simulink model "LugreFrictionTester"  (R2023b)
settings: Solver=ode4  StartTime=0.0  StopTime=t_final(end)  FixedStep=1e-3  RelTol=1e-3
undefined symbols (not defined in the file or in its folder): Aeff, m, xc, xc_dot
settings Model: Creator=snr  LastModifiedBy=snr

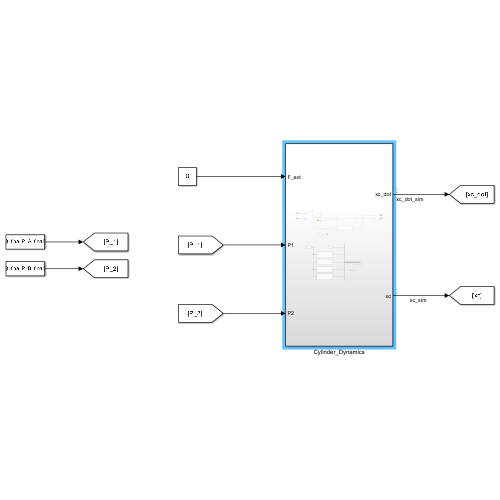
[thumbnail: Simulink's stored preview of the top-level diagram]
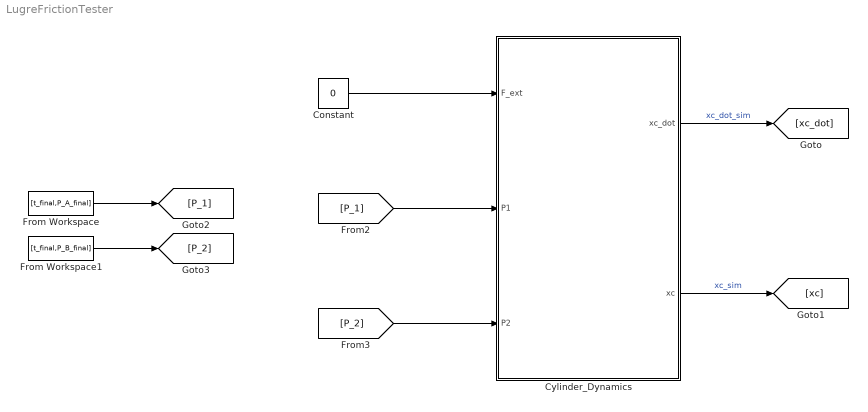
== system LugreFrictionTester ==
  Constant : Constant  Value=0  OutDataTypeStr=double
  Cylinder_Dynamics : Subsystem
  From Workspace : FromWorkspace  VariableName=[t_final,P_A_final]
  From Workspace1 : FromWorkspace  VariableName=[t_final,P_B_final]
  wires:
  Constant/1 -> Cylinder_Dynamics/1(F_ext)
  Cylinder_Dynamics/2(xc) -> [xc]  "xc_sim"
  [P_2] -> Cylinder_Dynamics/3(P2)
  [P_1] -> Cylinder_Dynamics/2(P1)
  Cylinder_Dynamics/1(xc_dot) -> [xc_dot]  "xc_dot_sim"
  From Workspace/1 -> [P_1]
  From Workspace1/1 -> [P_2]

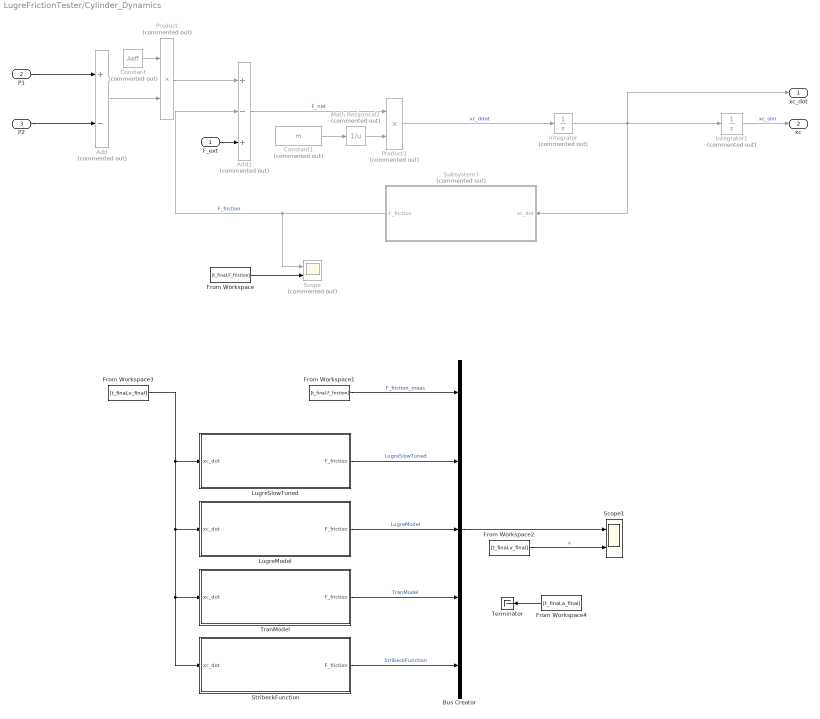
== system LugreFrictionTester/Cylinder_Dynamics ==
  F_ext : Inport  OutDataTypeStr=double
  P1 : Inport  Port=2  OutDataTypeStr=double
  P2 : Inport  Port=3  OutDataTypeStr=double
  Add : Sum  Commented=on  Inputs=+-
  Add1 : Sum  Commented=on  Inputs=+-+
  Bus Creator : BusCreator  Inputs=5
  Constant : Constant  Commented=on  Value=Aeff  OutDataTypeStr=double
  Constant1 : Constant  Commented=on  Value=m  OutDataTypeStr=double
  From Workspace : FromWorkspace  VariableName=[t_final,F_friction]
  From Workspace1 : FromWorkspace  VariableName=[t_final,F_friction]
  From Workspace2 : FromWorkspace  VariableName=[t_final,v_final]
  From Workspace3 : FromWorkspace  VariableName=[t_final,v_final]
  From Workspace4 : FromWorkspace  VariableName=[t_final,a_final]
  Integrator : Integrator  Commented=on  InitialCondition=xc_dot(1)
  Integrator1 : Integrator  Commented=on  InitialCondition=xc(1)
  LugreModel : Subsystem
  LugreSlowTuned : Subsystem
  Math Reciprocal2 : Math  Commented=on  Operator=reciprocal  SignedPower=on
  Product : Product  Commented=on
  Product1 : Product  Commented=on
  Scope : Scope  Commented=on  NumInputPorts=2
  Scope1 : Scope  NumInputPorts=2
  StribeckFunction : Subsystem
  Subsystem3 : Subsystem  Commented=on
  Terminator : Terminator
  TranModel : Subsystem
  xc_dot : Outport  OutDataTypeStr=double
  xc : Outport  Port=2  OutDataTypeStr=double
  wires:
  P2/1 -> Add/2
  P1/1 -> Add/1
  F_ext/1 -> Add1/3
  Integrator1/1 -> xc/1  "xc_sim"
  Add/1 -> Product/2
  Constant/1 -> Product/1
  Add1/1 -> Product1/1  "F_net"
  Constant1/1 -> Math Reciprocal2/1
  Math Reciprocal2/1 -> Product1/2
  Product1/1 -> Integrator/1  "xc_ddot"
  Integrator/1 -> Subsystem3/1(xc_dot), xc_dot/1, Integrator1/1
  Subsystem3/1(F_friction) -> Scope/1, Add1/2  "F_friction"
  Product/1 -> Add1/1
  From Workspace/1 -> Scope/2
  From Workspace3/1 -> StribeckFunction/1(xc_dot), TranModel/1(xc_dot), LugreModel/1(xc_dot), LugreSlowTuned/1(xc_dot)
  LugreModel/1(F_friction) -> Bus Creator/3  "LugreModel"
  TranModel/1(F_friction) -> Bus Creator/4  "TranModel"
  StribeckFunction/1(F_friction) -> Bus Creator/5  "StribeckFunction"
  From Workspace1/1 -> Bus Creator/1  "F_friction_meas"
  Bus Creator/1 -> Scope1/1
  From Workspace2/1 -> Scope1/2  "v"
  LugreSlowTuned/1(F_friction) -> Bus Creator/2  "LugreSlowTuned"
  From Workspace4/1 -> Terminator/1

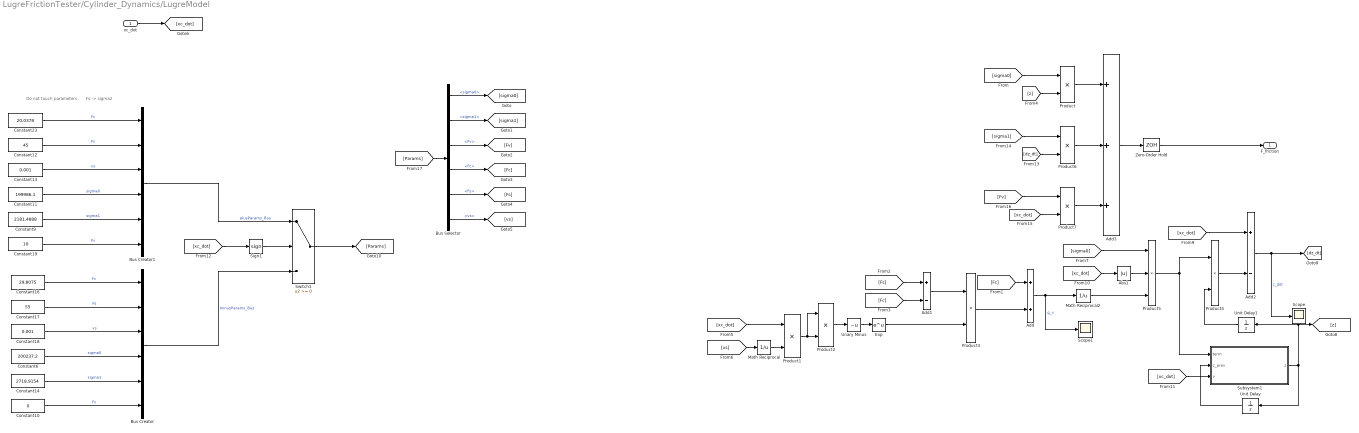
== system LugreFrictionTester/Cylinder_Dynamics/LugreModel ==
  note: Do not touch parameters
  note: Fv -> sigma2
  xc_dot : Inport
  Abs1 : Abs  SaturateOnIntegerOverflow=off
  Add : Sum
  Add1 : Sum  Inputs=+-
  Add2 : Sum  Inputs=+-
  Add3 : Sum  Inputs=+++
  Bus Selector : BusSelector  OutputSignals=sigma0,sigma1,Fv,Fc,Fs,vs
  Bus Creator : BusCreator  Inputs=6
  Bus Creator1 : BusCreator  Inputs=6
  Constant10 : Constant  Value=0  OutDataTypeStr=double
  Constant11 : Constant  Value=199986.1  OutDataTypeStr=double
  Constant12 : Constant  Value=45  OutDataTypeStr=double
  Constant13 : Constant  Value=0.001  OutDataTypeStr=double
  Constant14 : Constant  Value=2718.9154  OutDataTypeStr=double
  Constant16 : Constant  Value=29.8075  OutDataTypeStr=double
  Constant17 : Constant  Value=55  OutDataTypeStr=double
  Constant18 : Constant  Value=0.001  OutDataTypeStr=double
  Constant19 : Constant  Value=10  OutDataTypeStr=double
  Constant23 : Constant  Value=20.0378  OutDataTypeStr=double
  Constant6 : Constant  Value=200237.2  OutDataTypeStr=double
  Constant9 : Constant  Value=2181.4888  OutDataTypeStr=double
  Exp : Math  SignedPower=on
  Math Reciprocal : Math  Operator=reciprocal  SignedPower=on
  Math Reciprocal2 : Math  Operator=reciprocal  SignedPower=on
  Product{,1..4,6..7} (7 alike) : Product
  Product5 : Product  Inputs=3
  Scope : Scope
  Scope1 : Scope
  Sign1 : Signum
  Subsystem1 : Subsystem
  Switch1 : Switch  SaturateOnIntegerOverflow=off  InputSameDT=off
  Unary Minus : UnaryMinus
  Unit Delay : UnitDelay  SampleTime=-1  HasFrameUpgradeWarning=on
  Unit Delay1 : UnitDelay  SampleTime=-1  HasFrameUpgradeWarning=on
  Zero-Order Hold : ZeroOrderHold  SampleTime=1e-3
  F_friction : Outport
  wires:
  Zero-Order Hold/1 -> F_friction/1
  Product4/1 -> Add2/2
  Product5/1 -> Product4/1, Subsystem1/1(term)
  Unit Delay/1 -> Subsystem1/2(z_prev)
  Subsystem1/1(z) -> Unit Delay/1, Unit Delay1/1, [z]
  [xc_dot] -> Subsystem1/3(v)
  Unit Delay1/1 -> Product4/2
  [xc_dot] -> Add2/1
  Sign1/1 -> Switch1/2
  Add2/1 -> [dz_dt], Scope/1  "z_dot"
  Exp/1 -> Product3/2
  xc_dot/1 -> [xc_dot]
  Math Reciprocal2/1 -> Product5/3
  Bus Selector/6 -> [vs]  "<vs>"
  Bus Selector/5 -> [Fs]  "<Fs>"
  Bus Selector/4 -> [Fc]  "<Fc>"
  Bus Selector/3 -> [Fv]  "<Fv>"
  Bus Selector/2 -> [sigma1]  "<sigma1>"
  Bus Selector/1 -> [sigma0]  "<sigma0>"
  [Params] -> Bus Selector/1
  Switch1/1 -> [Params]
  Bus Creator/1 -> Switch1/3  "minusParams_Bus"
  Bus Creator1/1 -> Switch1/1  "plusParams_Bus"
  [xc_dot] -> Sign1/1
  Product3/1 -> Add/2
  [sigma0] -> Product/1
  [Fc] -> Add/1
  [Fs] -> Add1/1
  [Fc] -> Add1/2
  [vs] -> Math Reciprocal/1
  Math Reciprocal/1 -> Product1/2
  [xc_dot] -> Product1/1
  Product1/1 -> Product2/1, Product2/2
  Product2/1 -> Unary Minus/1
  Unary Minus/1 -> Exp/1
  Add1/1 -> Product3/1
  [xc_dot] -> Abs1/1
  Add/1 -> Scope1/1, Math Reciprocal2/1  "g_v"
  Abs1/1 -> Product5/2
  [sigma0] -> Product5/1
  [z] -> Product/2
  Product/1 -> Add3/1
  [sigma1] -> Product6/1
  [dz_dt] -> Product6/2
  [xc_dot] -> Product7/2
  [Fv] -> Product7/1
  Product6/1 -> Add3/2
  Product7/1 -> Add3/3
  Add3/1 -> Zero-Order Hold/1
  Constant23/1 -> Bus Creator1/1  "Fc"
  Constant19/1 -> Bus Creator1/6  "Fv"
  Constant11/1 -> Bus Creator1/4  "sigma0"
  Constant9/1 -> Bus Creator1/5  "sigma1"
  Constant16/1 -> Bus Creator/1  "Fc"
  Constant10/1 -> Bus Creator/6  "Fv"
  Constant6/1 -> Bus Creator/4  "sigma0"
  Constant14/1 -> Bus Creator/5  "sigma1"
  Constant17/1 -> Bus Creator/2  "Fs"
  Constant12/1 -> Bus Creator1/2  "Fs"
  Constant13/1 -> Bus Creator1/3  "vs"
  Constant18/1 -> Bus Creator/3  "vs"

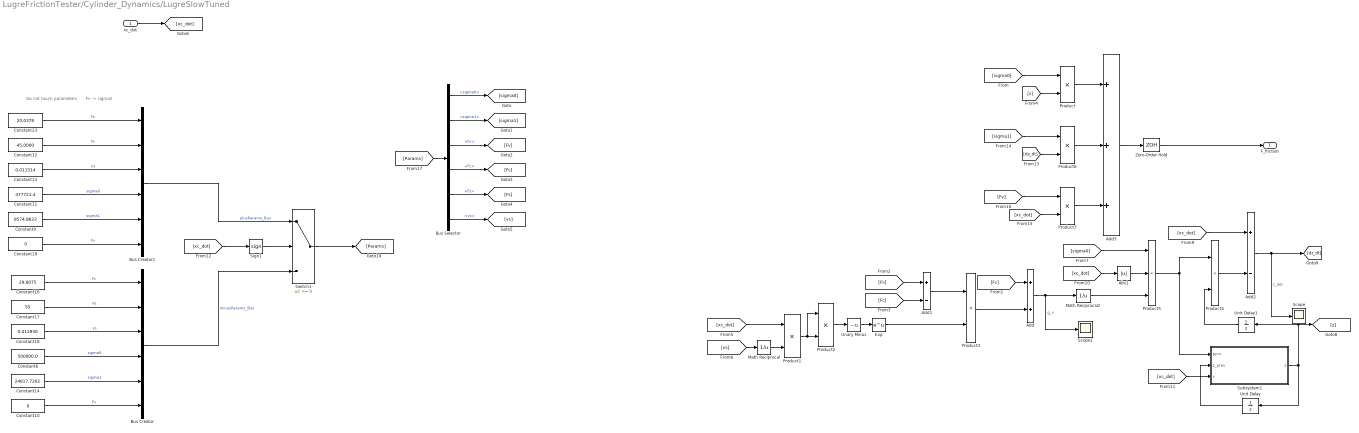
== system LugreFrictionTester/Cylinder_Dynamics/LugreSlowTuned ==
  note: Fv -> sigma2
  note: Do not touch parameters
  xc_dot : Inport
  Abs1 : Abs  SaturateOnIntegerOverflow=off
  Add : Sum
  Add1 : Sum  Inputs=+-
  Add2 : Sum  Inputs=+-
  Add3 : Sum  Inputs=+++
  Bus Selector : BusSelector  OutputSignals=sigma0,sigma1,Fv,Fc,Fs,vs
  Bus Creator : BusCreator  Inputs=6
  Bus Creator1 : BusCreator  Inputs=6
  Constant10 : Constant  Value=0  OutDataTypeStr=double
  Constant11 : Constant  Value=477721.4  OutDataTypeStr=double
  Constant12 : Constant  Value=45.0000  OutDataTypeStr=double
  Constant13 : Constant  Value=0.011514  OutDataTypeStr=double
  Constant14 : Constant  Value=24817.7202  OutDataTypeStr=double
  Constant16 : Constant  Value=29.8075  OutDataTypeStr=double
  Constant17 : Constant  Value=55  OutDataTypeStr=double
  Constant18 : Constant  Value=0.012930  OutDataTypeStr=double
  Constant19 : Constant  Value=0  OutDataTypeStr=double
  Constant23 : Constant  Value=20.0378  OutDataTypeStr=double
  Constant6 : Constant  Value=500000.0  OutDataTypeStr=double
  Constant9 : Constant  Value=8574.8623  OutDataTypeStr=double
  Exp : Math  SignedPower=on
  Math Reciprocal : Math  Operator=reciprocal  SignedPower=on
  Math Reciprocal2 : Math  Operator=reciprocal  SignedPower=on
  Product{,1..4,6..7} (7 alike) : Product
  Product5 : Product  Inputs=3
  Scope : Scope
  Scope1 : Scope
  Sign1 : Signum
  Subsystem1 : Subsystem
  Switch1 : Switch  SaturateOnIntegerOverflow=off  InputSameDT=off
  Unary Minus : UnaryMinus
  Unit Delay : UnitDelay  SampleTime=-1  HasFrameUpgradeWarning=on
  Unit Delay1 : UnitDelay  SampleTime=-1  HasFrameUpgradeWarning=on
  Zero-Order Hold : ZeroOrderHold  SampleTime=1e-3
  F_friction : Outport
  wires:
  Constant18/1 -> Bus Creator/3  "vs"
  Constant13/1 -> Bus Creator1/3  "vs"
  Constant12/1 -> Bus Creator1/2  "Fs"
  Constant17/1 -> Bus Creator/2  "Fs"
  Constant14/1 -> Bus Creator/5  "sigma1"
  Constant6/1 -> Bus Creator/4  "sigma0"
  Constant10/1 -> Bus Creator/6  "Fv"
  Constant16/1 -> Bus Creator/1  "Fc"
  Constant9/1 -> Bus Creator1/5  "sigma1"
  Constant11/1 -> Bus Creator1/4  "sigma0"
  Constant19/1 -> Bus Creator1/6  "Fv"
  Constant23/1 -> Bus Creator1/1  "Fc"
  Add3/1 -> Zero-Order Hold/1
  Product7/1 -> Add3/3
  Product6/1 -> Add3/2
  [Fv] -> Product7/1
  [xc_dot] -> Product7/2
  [dz_dt] -> Product6/2
  [sigma1] -> Product6/1
  Product/1 -> Add3/1
  [z] -> Product/2
  [sigma0] -> Product5/1
  Abs1/1 -> Product5/2
  Add/1 -> Math Reciprocal2/1, Scope1/1  "g_v"
  [xc_dot] -> Abs1/1
  Add1/1 -> Product3/1
  Unary Minus/1 -> Exp/1
  Product2/1 -> Unary Minus/1
  Product1/1 -> Product2/2, Product2/1
  [xc_dot] -> Product1/1
  Math Reciprocal/1 -> Product1/2
  [vs] -> Math Reciprocal/1
  [Fc] -> Add1/2
  [Fs] -> Add1/1
  [Fc] -> Add/1
  [sigma0] -> Product/1
  Product3/1 -> Add/2
  [xc_dot] -> Sign1/1
  Bus Creator1/1 -> Switch1/1  "plusParams_Bus"
  Bus Creator/1 -> Switch1/3  "minusParams_Bus"
  Switch1/1 -> [Params]
  [Params] -> Bus Selector/1
  Bus Selector/1 -> [sigma0]  "<sigma0>"
  Bus Selector/2 -> [sigma1]  "<sigma1>"
  Bus Selector/3 -> [Fv]  "<Fv>"
  Bus Selector/4 -> [Fc]  "<Fc>"
  Bus Selector/5 -> [Fs]  "<Fs>"
  Bus Selector/6 -> [vs]  "<vs>"
  Math Reciprocal2/1 -> Product5/3
  xc_dot/1 -> [xc_dot]
  Exp/1 -> Product3/2
  Add2/1 -> Scope/1, [dz_dt]  "z_dot"
  Sign1/1 -> Switch1/2
  [xc_dot] -> Add2/1
  Unit Delay1/1 -> Product4/2
  [xc_dot] -> Subsystem1/3(v)
  Subsystem1/1(z) -> [z], Unit Delay1/1, Unit Delay/1
  Unit Delay/1 -> Subsystem1/2(z_prev)
  Product5/1 -> Subsystem1/1(term), Product4/1
  Product4/1 -> Add2/2
  Zero-Order Hold/1 -> F_friction/1

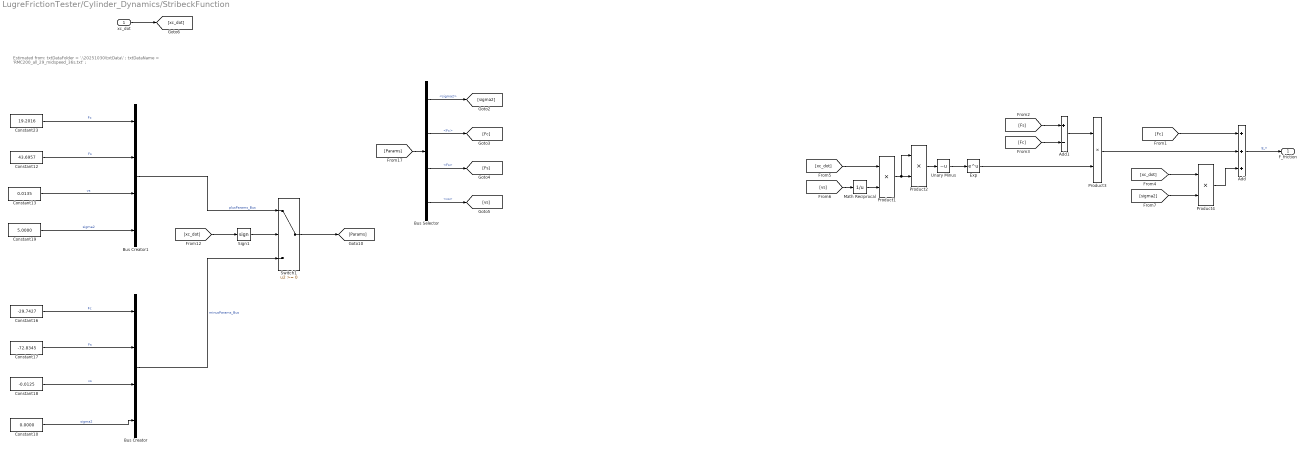
== system LugreFrictionTester/Cylinder_Dynamics/StribeckFunction ==
  note: Estimated from:
      |
      | txtDataFolder = '.\20251030\txtData\' ;
      | txtDataName = 'RMC200_all_29_midspeed_36s.txt' ;
  xc_dot : Inport
  Add : Sum  Inputs=+++
  Add1 : Sum  Inputs=+-
  Bus Selector : BusSelector  OutputSignals=sigma2,Fc,Fs,vs
  Bus Creator : BusCreator  Inputs=4
  Bus Creator1 : BusCreator  Inputs=4
  Constant10 : Constant  Value=0.0000  OutDataTypeStr=double
  Constant12 : Constant  Value=43.6957  OutDataTypeStr=double
  Constant13 : Constant  Value=0.0135  OutDataTypeStr=double
  Constant16 : Constant  Value=-29.7427  OutDataTypeStr=double
  Constant17 : Constant  Value=-72.8345  OutDataTypeStr=double
  Constant18 : Constant  Value=-0.0125  OutDataTypeStr=double
  Constant19 : Constant  Value=5.0000  OutDataTypeStr=double
  Constant23 : Constant  Value=19.2016  OutDataTypeStr=double
  Exp : Math  SignedPower=on
  Math Reciprocal : Math  Operator=reciprocal  SignedPower=on
  Product{1..4} (4 alike) : Product
  Sign1 : Signum
  Switch1 : Switch  SaturateOnIntegerOverflow=off  InputSameDT=off
  Unary Minus : UnaryMinus
  F_friction : Outport
  wires:
  Sign1/1 -> Switch1/2
  Exp/1 -> Product3/2
  xc_dot/1 -> [xc_dot]
  Bus Selector/4 -> [vs]  "<vs>"
  Bus Selector/3 -> [Fs]  "<Fs>"
  Bus Selector/2 -> [Fc]  "<Fc>"
  Bus Selector/1 -> [sigma2]  "<sigma2>"
  [Params] -> Bus Selector/1
  Switch1/1 -> [Params]
  Bus Creator/1 -> Switch1/3  "minusParams_Bus"
  Bus Creator1/1 -> Switch1/1  "plusParams_Bus"
  [xc_dot] -> Sign1/1
  Product3/1 -> Add/2
  [Fc] -> Add/1
  [Fs] -> Add1/1
  [Fc] -> Add1/2
  [vs] -> Math Reciprocal/1
  Math Reciprocal/1 -> Product1/2
  [xc_dot] -> Product1/1
  Product1/1 -> Product2/1, Product2/2
  Product2/1 -> Unary Minus/1
  Unary Minus/1 -> Exp/1
  Add1/1 -> Product3/1
  Add/1 -> F_friction/1  "g_v"
  Constant23/1 -> Bus Creator1/1  "Fc"
  Constant19/1 -> Bus Creator1/4  "sigma2"
  Constant16/1 -> Bus Creator/1  "Fc"
  Constant10/1 -> Bus Creator/4  "sigma2"
  Constant17/1 -> Bus Creator/2  "Fs"
  Constant12/1 -> Bus Creator1/2  "Fs"
  Constant13/1 -> Bus Creator1/3  "vs"
  Constant18/1 -> Bus Creator/3  "vs"
  [xc_dot] -> Product4/1
  [sigma2] -> Product4/2
  Product4/1 -> Add/3

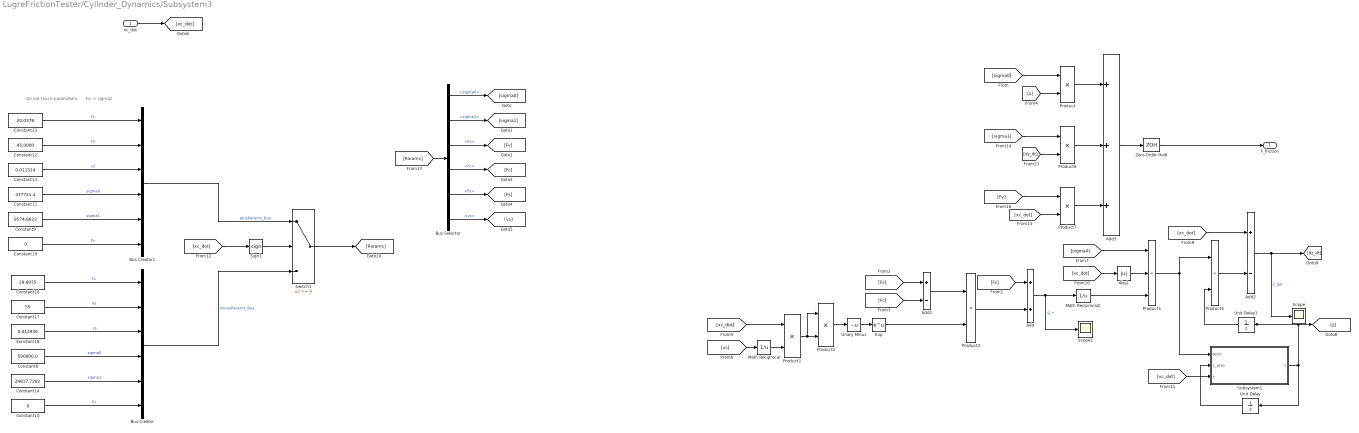
== system LugreFrictionTester/Cylinder_Dynamics/Subsystem3 ==
  note: Do not touch parameters
  note: Fv -> sigma2
  xc_dot : Inport
  Abs1 : Abs  SaturateOnIntegerOverflow=off
  Add : Sum
  Add1 : Sum  Inputs=+-
  Add2 : Sum  Inputs=+-
  Add3 : Sum  Inputs=+++
  Bus Selector : BusSelector  OutputSignals=sigma0,sigma1,Fv,Fc,Fs,vs
  Bus Creator : BusCreator  Inputs=6
  Bus Creator1 : BusCreator  Inputs=6
  Constant10 : Constant  Value=0  OutDataTypeStr=double
  Constant11 : Constant  Value=477721.4  OutDataTypeStr=double
  Constant12 : Constant  Value=45.0000  OutDataTypeStr=double
  Constant13 : Constant  Value=0.011514  OutDataTypeStr=double
  Constant14 : Constant  Value=24817.7202  OutDataTypeStr=double
  Constant16 : Constant  Value=29.8075  OutDataTypeStr=double
  Constant17 : Constant  Value=55  OutDataTypeStr=double
  Constant18 : Constant  Value=0.012930  OutDataTypeStr=double
  Constant19 : Constant  Value=0  OutDataTypeStr=double
  Constant23 : Constant  Value=20.0378  OutDataTypeStr=double
  Constant6 : Constant  Value=500000.0  OutDataTypeStr=double
  Constant9 : Constant  Value=8574.8623  OutDataTypeStr=double
  Exp : Math  SignedPower=on
  Math Reciprocal : Math  Operator=reciprocal  SignedPower=on
  Math Reciprocal2 : Math  Operator=reciprocal  SignedPower=on
  Product{,1..4,6..7} (7 alike) : Product
  Product5 : Product  Inputs=3
  Scope : Scope
  Scope1 : Scope
  Sign1 : Signum
  Subsystem1 : Subsystem
  Switch1 : Switch  SaturateOnIntegerOverflow=off  InputSameDT=off
  Unary Minus : UnaryMinus
  Unit Delay : UnitDelay  SampleTime=-1  HasFrameUpgradeWarning=on
  Unit Delay1 : UnitDelay  SampleTime=-1  HasFrameUpgradeWarning=on
  Zero-Order Hold : ZeroOrderHold  SampleTime=1e-3
  F_friction : Outport
  wires:
  Zero-Order Hold/1 -> F_friction/1
  Product4/1 -> Add2/2
  Product5/1 -> Product4/1, Subsystem1/1(term)
  Unit Delay/1 -> Subsystem1/2(z_prev)
  Subsystem1/1(z) -> Unit Delay/1, Unit Delay1/1, [z]
  [xc_dot] -> Subsystem1/3(v)
  Unit Delay1/1 -> Product4/2
  [xc_dot] -> Add2/1
  Sign1/1 -> Switch1/2
  Add2/1 -> [dz_dt], Scope/1  "z_dot"
  Exp/1 -> Product3/2
  xc_dot/1 -> [xc_dot]
  Math Reciprocal2/1 -> Product5/3
  Bus Selector/6 -> [vs]  "<vs>"
  Bus Selector/5 -> [Fs]  "<Fs>"
  Bus Selector/4 -> [Fc]  "<Fc>"
  Bus Selector/3 -> [Fv]  "<Fv>"
  Bus Selector/2 -> [sigma1]  "<sigma1>"
  Bus Selector/1 -> [sigma0]  "<sigma0>"
  [Params] -> Bus Selector/1
  Switch1/1 -> [Params]
  Bus Creator/1 -> Switch1/3  "minusParams_Bus"
  Bus Creator1/1 -> Switch1/1  "plusParams_Bus"
  [xc_dot] -> Sign1/1
  Product3/1 -> Add/2
  [sigma0] -> Product/1
  [Fc] -> Add/1
  [Fs] -> Add1/1
  [Fc] -> Add1/2
  [vs] -> Math Reciprocal/1
  Math Reciprocal/1 -> Product1/2
  [xc_dot] -> Product1/1
  Product1/1 -> Product2/1, Product2/2
  Product2/1 -> Unary Minus/1
  Unary Minus/1 -> Exp/1
  Add1/1 -> Product3/1
  [xc_dot] -> Abs1/1
  Add/1 -> Scope1/1, Math Reciprocal2/1  "g_v"
  Abs1/1 -> Product5/2
  [sigma0] -> Product5/1
  [z] -> Product/2
  Product/1 -> Add3/1
  [sigma1] -> Product6/1
  [dz_dt] -> Product6/2
  [xc_dot] -> Product7/2
  [Fv] -> Product7/1
  Product6/1 -> Add3/2
  Product7/1 -> Add3/3
  Add3/1 -> Zero-Order Hold/1
  Constant23/1 -> Bus Creator1/1  "Fc"
  Constant19/1 -> Bus Creator1/6  "Fv"
  Constant11/1 -> Bus Creator1/4  "sigma0"
  Constant9/1 -> Bus Creator1/5  "sigma1"
  Constant16/1 -> Bus Creator/1  "Fc"
  Constant10/1 -> Bus Creator/6  "Fv"
  Constant6/1 -> Bus Creator/4  "sigma0"
  Constant14/1 -> Bus Creator/5  "sigma1"
  Constant17/1 -> Bus Creator/2  "Fs"
  Constant12/1 -> Bus Creator1/2  "Fs"
  Constant13/1 -> Bus Creator1/3  "vs"
  Constant18/1 -> Bus Creator/3  "vs"

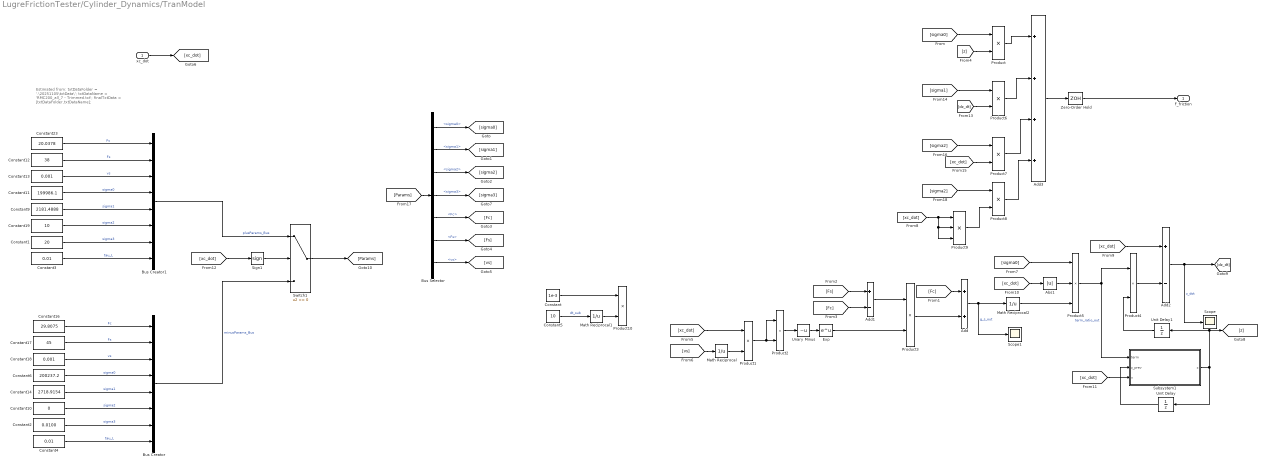
== system LugreFrictionTester/Cylinder_Dynamics/TranModel ==
  note: Estimated from:
      |
      | txtDataFolder = '.\20251105\txtData\';
      | txtDataName = 'RMC200_all_7 - Trimmed.txt';
      | finalTxtData = [txtDataFolder,txtDataName];
  xc_dot : Inport
  Abs1 : Abs  SaturateOnIntegerOverflow=off
  Add : Sum
  Add1 : Sum  Inputs=+-
  Add2 : Sum  Inputs=+-
  Add3 : Sum  Inputs=++++
  Bus Selector : BusSelector  OutputSignals=sigma0,sigma1,sigma2,sigma3,Fc,Fs,vs
  Bus Creator : BusCreator  Inputs=8
  Bus Creator1 : BusCreator  Inputs=8
  Constant : Constant  Value=1e-3
  Constant1 : Constant  Value=20  OutDataTypeStr=double
  Constant10 : Constant  Value=0  OutDataTypeStr=double
  Constant11 : Constant  Value=199986.1  OutDataTypeStr=double
  Constant12 : Constant  Value=38  OutDataTypeStr=double
  Constant13 : Constant  Value=0.001  OutDataTypeStr=double
  Constant14 : Constant  Value=2718.9154  OutDataTypeStr=double
  Constant16 : Constant  Value=29.8075  OutDataTypeStr=double
  Constant17 : Constant  Value=45  OutDataTypeStr=double
  Constant18 : Constant  Value=0.001  OutDataTypeStr=double
  Constant19 : Constant  Value=10  OutDataTypeStr=double
  Constant2 : Constant  Value=0.0100  OutDataTypeStr=double
  Constant23 : Constant  Value=20.0378  OutDataTypeStr=double
  Constant3 : Constant  Value=0.01  OutDataTypeStr=double
  Constant4 : Constant  Value=0.01  OutDataTypeStr=double
  Constant5 : Constant  Value=10
  Constant6 : Constant  Value=200237.2  OutDataTypeStr=double
  Constant9 : Constant  Value=2181.4888  OutDataTypeStr=double
  Exp : Math  SignedPower=on
  Math Reciprocal : Math  Operator=reciprocal  SignedPower=on
  Math Reciprocal1 : Math  Operator=reciprocal  SignedPower=on
  Math Reciprocal2 : Math  Operator=reciprocal  SignedPower=on
  Product{,1..4,6..8,10} (9 alike) : Product
  Product5 : Product  Inputs=3
  Product9 : Product  Inputs=3
  Scope : Scope
  Scope1 : Scope
  Sign1 : Signum
  Subsystem1 : Subsystem
  Switch1 : Switch  SaturateOnIntegerOverflow=off  InputSameDT=off
  Unary Minus : UnaryMinus
  Unit Delay : UnitDelay  SampleTime=-1  HasFrameUpgradeWarning=on
  Unit Delay1 : UnitDelay  SampleTime=-1  HasFrameUpgradeWarning=on
  Zero-Order Hold : ZeroOrderHold  SampleTime=1e-3
  F_friction : Outport
  wires:
  Constant18/1 -> Bus Creator/3  "vs"
  Constant13/1 -> Bus Creator1/3  "vs"
  Constant12/1 -> Bus Creator1/2  "Fs"
  Constant17/1 -> Bus Creator/2  "Fs"
  Constant14/1 -> Bus Creator/5  "sigma1"
  Constant6/1 -> Bus Creator/4  "sigma0"
  Constant10/1 -> Bus Creator/6  "sigma2"
  Constant16/1 -> Bus Creator/1  "Fc"
  Constant9/1 -> Bus Creator1/5  "sigma1"
  Constant11/1 -> Bus Creator1/4  "sigma0"
  Constant19/1 -> Bus Creator1/6  "sigma2"
  Constant23/1 -> Bus Creator1/1  "Fc"
  Add3/1 -> Zero-Order Hold/1
  Product7/1 -> Add3/3
  Product6/1 -> Add3/2
  [sigma2] -> Product7/1
  [xc_dot] -> Product7/2
  [dz_dt] -> Product6/2
  [sigma1] -> Product6/1
  Product/1 -> Add3/1
  [z] -> Product/2
  [sigma0] -> Product5/1
  Abs1/1 -> Product5/2
  Add/1 -> Math Reciprocal2/1, Scope1/1  "g_s_out"
  [xc_dot] -> Abs1/1
  Add1/1 -> Product3/1
  Unary Minus/1 -> Exp/1
  Product2/1 -> Unary Minus/1
  Product1/1 -> Product2/2, Product2/1
  [xc_dot] -> Product1/1
  Math Reciprocal/1 -> Product1/2
  [vs] -> Math Reciprocal/1
  [Fc] -> Add1/2
  [Fs] -> Add1/1
  [Fc] -> Add/1
  [sigma0] -> Product/1
  Product3/1 -> Add/2
  [xc_dot] -> Sign1/1
  Bus Creator1/1 -> Switch1/1  "plusParams_Bus"
  Bus Creator/1 -> Switch1/3  "minusParams_Bus"
  Switch1/1 -> [Params]
  [Params] -> Bus Selector/1
  Bus Selector/1 -> [sigma0]  "<sigma0>"
  Bus Selector/2 -> [sigma1]  "<sigma1>"
  Bus Selector/3 -> [sigma2]  "<sigma2>"
  Bus Selector/5 -> [Fc]  "<Fc>"
  Bus Selector/6 -> [Fs]  "<Fs>"
  Bus Selector/7 -> [vs]  "<vs>"
  Math Reciprocal2/1 -> Product5/3
  xc_dot/1 -> [xc_dot]
  Exp/1 -> Product3/2
  Add2/1 -> Scope/1, [dz_dt]  "z_dot"
  Sign1/1 -> Switch1/2
  [xc_dot] -> Add2/1
  Unit Delay1/1 -> Product4/2
  [xc_dot] -> Subsystem1/3(v)
  Subsystem1/1(z) -> [z], Unit Delay1/1, Unit Delay/1
  Unit Delay/1 -> Subsystem1/2(z_prev)
  Product5/1 -> Subsystem1/1(term), Product4/1  "term_ratio_out"
  Product4/1 -> Add2/2
  Zero-Order Hold/1 -> F_friction/1
  Constant1/1 -> Bus Creator1/7  "sigma3"
  Constant2/1 -> Bus Creator/7  "sigma3"
  Constant3/1 -> Bus Creator1/8  "tau_L"
  Constant4/1 -> Bus Creator/8  "tau_L"
  [sigma2] -> Product8/1
  Product8/1 -> Add3/4
  [xc_dot] -> Product9/2, Product9/3, Product9/1
  Product9/1 -> Product8/2
  Bus Selector/4 -> [sigma3]  "<sigma3>"
  Constant5/1 -> Math Reciprocal1/1  "dt_sub"
  Math Reciprocal1/1 -> Product10/2
  Constant/1 -> Product10/1

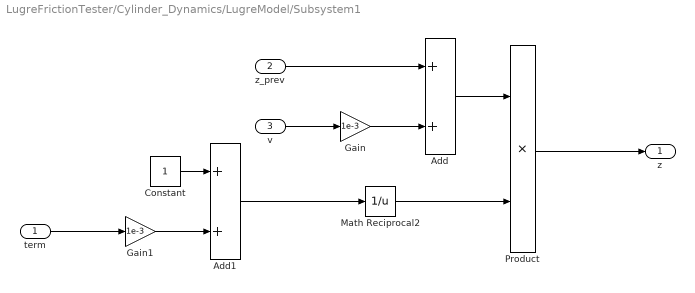
== system LugreFrictionTester/Cylinder_Dynamics/LugreModel/Subsystem1 ==
  term : Inport
  z_prev : Inport  Port=2
  v : Inport  Port=3
  Add : Sum
  Add1 : Sum
  Constant : Constant
  Gain : Gain  Gain=1e-3
  Gain1 : Gain  Gain=1e-3
  Math Reciprocal2 : Math  Operator=reciprocal  SignedPower=on
  Product : Product
  z : Outport
  wires:
  Product/1 -> z/1
  Math Reciprocal2/1 -> Product/2
  Add1/1 -> Math Reciprocal2/1
  Constant/1 -> Add1/1
  Gain1/1 -> Add1/2
  Add/1 -> Product/1
  Gain/1 -> Add/2
  v/1 -> Gain/1
  z_prev/1 -> Add/1
  term/1 -> Gain1/1

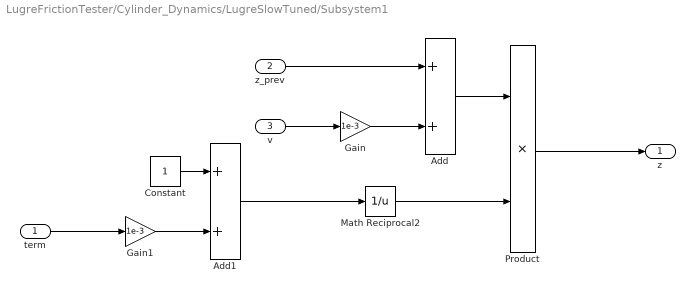
== system LugreFrictionTester/Cylinder_Dynamics/LugreSlowTuned/Subsystem1 ==
  term : Inport
  z_prev : Inport  Port=2
  v : Inport  Port=3
  Add : Sum
  Add1 : Sum
  Constant : Constant
  Gain : Gain  Gain=1e-3
  Gain1 : Gain  Gain=1e-3
  Math Reciprocal2 : Math  Operator=reciprocal  SignedPower=on
  Product : Product
  z : Outport
  wires:
  term/1 -> Gain1/1
  z_prev/1 -> Add/1
  v/1 -> Gain/1
  Gain/1 -> Add/2
  Add/1 -> Product/1
  Gain1/1 -> Add1/2
  Constant/1 -> Add1/1
  Add1/1 -> Math Reciprocal2/1
  Math Reciprocal2/1 -> Product/2
  Product/1 -> z/1

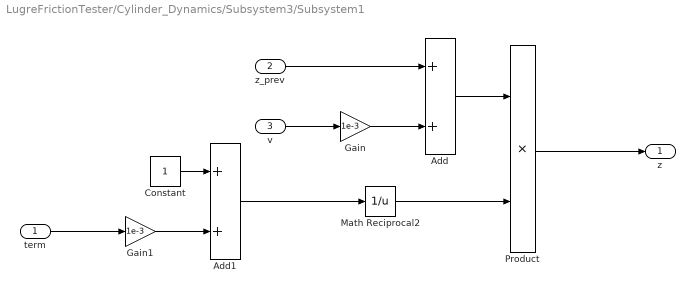
== system LugreFrictionTester/Cylinder_Dynamics/Subsystem3/Subsystem1 ==
  term : Inport
  z_prev : Inport  Port=2
  v : Inport  Port=3
  Add : Sum
  Add1 : Sum
  Constant : Constant
  Gain : Gain  Gain=1e-3
  Gain1 : Gain  Gain=1e-3
  Math Reciprocal2 : Math  Operator=reciprocal  SignedPower=on
  Product : Product
  z : Outport
  wires:
  Product/1 -> z/1
  Math Reciprocal2/1 -> Product/2
  Add1/1 -> Math Reciprocal2/1
  Constant/1 -> Add1/1
  Gain1/1 -> Add1/2
  Add/1 -> Product/1
  Gain/1 -> Add/2
  v/1 -> Gain/1
  z_prev/1 -> Add/1
  term/1 -> Gain1/1

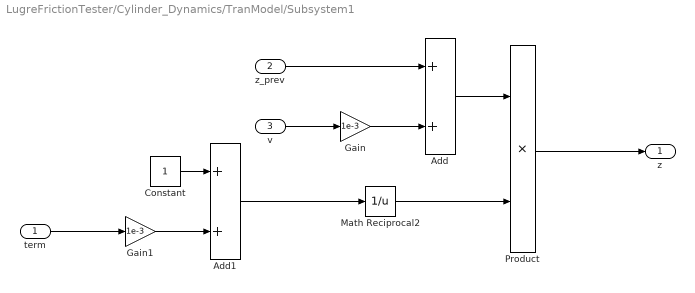
== system LugreFrictionTester/Cylinder_Dynamics/TranModel/Subsystem1 ==
  term : Inport
  z_prev : Inport  Port=2
  v : Inport  Port=3
  Add : Sum
  Add1 : Sum
  Constant : Constant
  Gain : Gain  Gain=1e-3
  Gain1 : Gain  Gain=1e-3
  Math Reciprocal2 : Math  Operator=reciprocal  SignedPower=on
  Product : Product
  z : Outport
  wires:
  term/1 -> Gain1/1
  z_prev/1 -> Add/1
  v/1 -> Gain/1
  Gain/1 -> Add/2
  Add/1 -> Product/1
  Gain1/1 -> Add1/2
  Constant/1 -> Add1/1
  Add1/1 -> Math Reciprocal2/1
  Math Reciprocal2/1 -> Product/2
  Product/1 -> z/1
